simulink model "faultSimulation"  (R2024a)
settings: Solver=VariableStepAuto  StartTime=0.0  StopTime=0.5  RelTol=1e-3
libraries: spsThreePhaseVIMeasurementLib x2, spsRMSLib x2, spsDistributedParametersLineLib x2, spsSequenceAnalyzerLib x2, spsThreePhaseSeriesRLCLoadLib x1, spsThreePhaseSourceLib x1, spsThreePhaseTransformerTwoWindingsLib x1, spsThreePhaseFaultLib x1, spspowerguiLib x1
settings Model: Creator=Subash  LastModifiedBy=subed
settings DataIOCC: SaveFormat=StructureWithTime  SaveState=on  ReturnWorkspaceOutputs=off
settings OptimizationCC: ReuseModelBlockBuffer=off
settings RTWCC: GPUComputeCapability=3.5

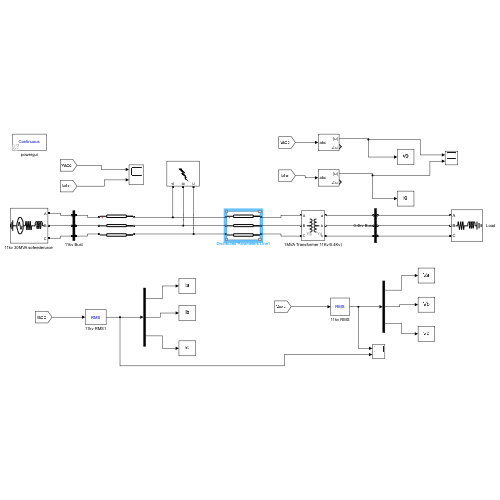
[thumbnail: Simulink's stored preview of the top-level diagram]
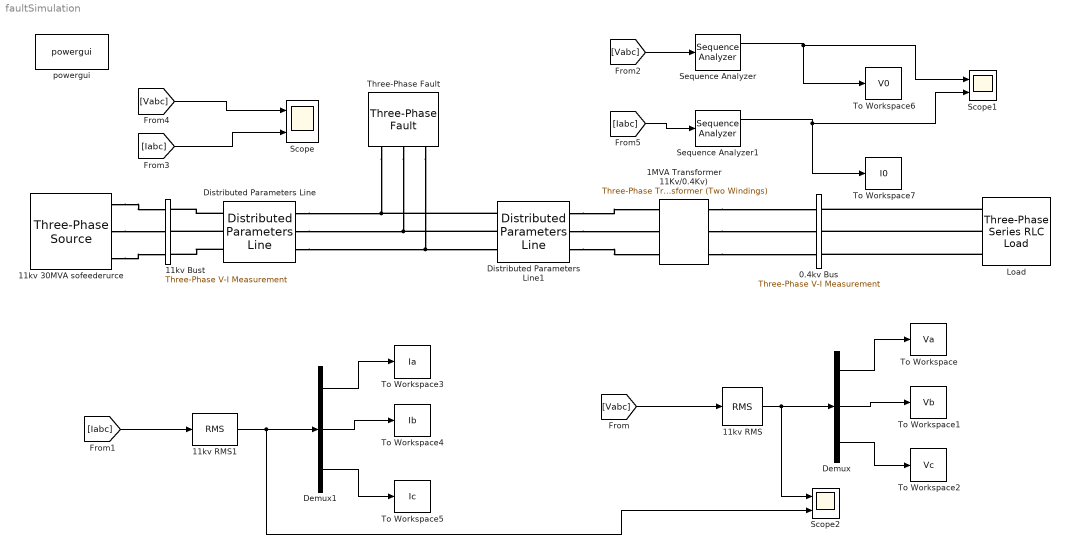
== system faultSimulation ==
  " Load" : spsThreePhaseSeriesRLCLoadLib/Three-Phase Series RLC Load  LConnTagsString=A|B|C  Configuration=Y (grounded)  NominalVoltage=11000  Vabc=[1e3 1e3 1e3]  Vabcp=[1e3 1e3 1e3]  NominalFrequency=50  UnbalancedPower=off  ActivePower=11e3  InductivePower=1  CapacitivePower=0  Pabc=[10e3 9e3 11e3]  QLabc=[100 90 110]  QCabc=0  Pabcp=[10e3 9e3 11e3]  QLabcp=[100 90 110]  QCabcp=[100 90 110]  Measurements=None  LoadType=constant Z
  0.4kv Bus : spsThreePhaseVIMeasurementLib/Three-Phase V-I Measurement  VoltageMeasurement=no  SetLabelV=off  LabelV=Vabc  Vpu=off  VpuLL=off  CurrentMeasurement=no  SetLabelI=off  LabelI=Iabc  Ipu=off  Pbase=100e6  Vbase=500e3  OutputType=Complex  PhasorSimulation=off  PSBequivalent=0
  "11kv 30MVA sofeederurce " : spsThreePhaseSourceLib/Three-Phase Source  InternalConnection=Yg  VoltagePhases=off  Voltage=11e3  PhaseAngle=0  Voltage_phases=[25e3 25e3 25e3]/sqrt(3)  PhaseAngles_phases=[0 -120 +120]  Frequency=50  NonIdealSource=on  SpecifyImpedance=off  Resistance=0.8929  Inductance=16.58e-3  ShortCircuitLevel=100e6  BaseVoltage=25e3  XRratio=7  BusType=PV  Pref=30e6  Qref=0  Prefabc=[10e3, 10e3, 10e3]  Qrefabc=[0, 0, 0]  Qmin=-inf  Qmax=inf
  11kv Bust : spsThreePhaseVIMeasurementLib/Three-Phase V-I Measurement  VoltageMeasurement=phase-to-ground  SetLabelV=on  LabelV=Vabc  Vpu=off  VpuLL=off  CurrentMeasurement=yes  SetLabelI=on  LabelI=Iabc  Ipu=off  Pbase=100e6  Vbase=500e3  OutputType=Complex  PhasorSimulation=off  PSBequivalent=0
  11kv RMS : spsRMSLib/RMS  TrueRMS=on  Freq=50  RMSInit=11e3  Ts=0
  11kv RMS1 : spsRMSLib/RMS  TrueRMS=on  Freq=50  RMSInit=11e3  Ts=0
  1MVA Transformer 11Kv/0.4Kv) : spsThreePhaseTransformerTwoWindingsLib/Three-Phase Transformer (Two Windings)  Winding1Connection=Yg  Winding2Connection=Yg  CoreType=Three single-phase transformers  SetSaturation=off  Hysteresis=off  DataFile='hysteresis'  SetInitialFlux=off  Measurements=None  UNITS=pu  NominalPower=[ 250e6 , 50 ]  Winding1=[ 11e3 , 0.002 , 0.08 ]  Winding2=[ 0.4e3 , 0.002 , 0.08 ]  Rm=500  Lm=500  L0=0.5  Saturation=[ 0,0 ; 0.0024,1.2 ; 1.0,1.52 ]  InitialFluxes=[0.8 -0.8 0.69999]  BreakLoop=off  DiscreteSolver=Trapezoidal iterative  DataType=off  TransfoNumber=1
  Demux : Demux  Outputs=3
  Demux1 : Demux  Outputs=3
  Distributed Parameters Line : spsDistributedParametersLineLib/Distributed Parameters Line  Phases=3  Length=10  Frequency=50  Resistance=[0.01273 0.3864]  Inductance="[0.9337e-3  4.1264e-3]"  Capacitance=[12.74e-9 7.751e-9]  x1=[4.29007792811563e-12 11003.1893836905 11003.1893836905;314.159265358979 314.159265358979 314.159265358979;2.11162862981672 0.512613974625824 -1.05818235216907]  x2=[2.73605273041382e-11 11004.416576192 11004.416576192;314.159265358979 314.159265358979 314.159265358979;2.85465814848236 0.512554423166818 -1.05824190362808]  x3=[2.29013626664532e-12 40.4303240016951 40.430324001691;314.159265358979 314.159265358979 314.159265358979;1.52130621419638 0.496602964655876 -1.07419336213898]  x4=[1.63728049127687e-12 40.8398210682543 40.8398210682578;314.159265358979 314.159265358979 314.159265358979;-1.19077244951278 0.517623004877797 -1.05317332191716]  x5=5.65541566995743e-05  V1=[4.29e-12 1.1e+04 1.1e+04;314.2 314.2 314.2;2.112 0.5126 -1.058]  V2=[2.736e-11 1.1e+04 1.1e+04;314.2 314.2 314.2;2.855 0.5126 -1.058]  I1=[2.29e-12 40.43 40.43;314.2 314.2 314.2;1.521 0.4966 -1.074]  I2=[1.637e-12 40.84 40.84;314.2 314.2 314.2;-1.191 0.5176 -1.053]  nHarmo=1  Measurements=None  Decoupling=off  VsMag0=0  VrMag0=0  VsAngle0=0  VrAngle0=0  IsMag0=0  IrMag0=0  IsAngle0=0  IrAngle0=0
      settings: LibrarySourceBlock=sps_lib/Power Grid Elements/Distributed Parameters Line
  Distributed Parameters Line1 : spsDistributedParametersLineLib/Distributed Parameters Line  Phases=3  Length=15  Frequency=50  Resistance=[0.01273 0.3864]  Inductance="[0.9337e-3  4.1264e-3]"  Capacitance=[12.74e-9 7.751e-9]  x1=[2.73605273041382e-11 11004.416576192 11004.416576192;314.159265358979 314.159265358979 314.159265358979;2.86354165464323 0.517972039807862 -1.05282428698704]  x2=[2.80656861363413e-11 11004.5464151717 11004.5464151717;314.159265358979 314.159265358979 314.159265358979;2.66181528844822 0.51794564452879 -1.05285068226611]  x3=[1.0173475413593e-12 40.4483736960803 40.4483736960805;314.159265358979 314.159265358979 314.159265358979;-2.35891284635151 0.512853803783494 -1.05794252301145]  x4=[1.45823347498536e-12 40.8359622190735 40.8359622190726;314.159265358979 314.159265358979 314.159265358979;3.13298239483697 0.517623203319764 -1.05317312347505]  x5=2.82770783497871e-05  V1=[2.736e-11 1.1e+04 1.1e+04;314.2 314.2 314.2;2.864 0.518 -1.053]  V2=[2.807e-11 1.1e+04 1.1e+04;314.2 314.2 314.2;2.662 0.5179 -1.053]  I1=[1.017e-12 40.45 40.45;314.2 314.2 314.2;-2.359 0.5129 -1.058]  I2=[1.458e-12 40.84 40.84;314.2 314.2 314.2;3.133 0.5176 -1.053]  nHarmo=1  Measurements=None  Decoupling=off  VsMag0=0  VrMag0=0  VsAngle0=0  VrAngle0=0  IsMag0=0  IrMag0=0  IsAngle0=0  IrAngle0=0
      settings: LibrarySourceBlock=sps_lib/Power Grid Elements/Distributed Parameters Line
  Scope : Scope  NumInputPorts=2
  Scope1 : Scope  NumInputPorts=2
  Scope2 : Scope  NumInputPorts=2
  Sequence Analyzer : spsSequenceAnalyzerLib/Sequence Analyzer  Freq=50  n=1  seq=Zero  InInit=[1, 0]  Ts=0
      settings: LibrarySourceBlock=sps_lib/Sensors and Measurements/Sequence Analyzer
  Sequence Analyzer1 : spsSequenceAnalyzerLib/Sequence Analyzer  Freq=50  n=1  seq=Zero  InInit=[1, 0]  Ts=0
      settings: LibrarySourceBlock=sps_lib/Sensors and Measurements/Sequence Analyzer
  Three-Phase Fault : spsThreePhaseFaultLib/Three-Phase Fault  InitialStates=0  FaultA=on  FaultB=off  FaultC=off  GroundFault=on  SwitchTimes=[0.2 0.3]  External=off  SwitchStatus=NaN  FaultResistance=0.001  GroundResistance=0.01  SnubberResistance=1e6  SnubberCapacitance=inf  Measurements=Fault voltages and currents
  To Workspace : ToWorkspace  VariableName=Va  SampleTime=-1
      settings: MaxDataPoints=15
  To Workspace1 : ToWorkspace  VariableName=Vb  SampleTime=-1
      settings: MaxDataPoints=15
  To Workspace2 : ToWorkspace  VariableName=Vc  SampleTime=-1
      settings: MaxDataPoints=15
  To Workspace3 : ToWorkspace  VariableName=Ia  SampleTime=-1
      settings: MaxDataPoints=15
  To Workspace4 : ToWorkspace  VariableName=Ib  SampleTime=-1
      settings: MaxDataPoints=15
  To Workspace5 : ToWorkspace  VariableName=Ic  SampleTime=-1
      settings: MaxDataPoints=15
  To Workspace6 : ToWorkspace  VariableName=V0  SampleTime=-1
      settings: MaxDataPoints=15
  To Workspace7 : ToWorkspace  VariableName=I0  SampleTime=-1
      settings: MaxDataPoints=15
  powergui : spspowerguiLib/powergui  Priority=1  SimulationMode=Continuous  SampleTime=50e-6  frequency=60  Iterations=50  frequencyindice=50  Pbase=100e6  ErrMax=1e-4  UnitsV=kV  UnitsW=MW  buscounter=0  FunctionMessages=off  echomessages=off  EnableUseOfTLC=off  CurrentSourceSwitches=off  DisableSnubberDevices=off  DisableRonSwitches=off  DisableVfSwitches=off  DisplayEquations=off  AutomaticDiscreteSolvers=off  SolverType=Tustin/Backward Euler (TBE)  Interpol=off  ExternalGateDelay=off  methode=off  Ts=100  x0status=blocks  SPID=on  SwTol=0  HookPort=off  NonlinearTolerance=1e-4  nMaxIteration=100  ContinueOnMaxIteration=off  RestoreLinks=warning  ResistiveCurrentMeasurement=off  Frange=[0:2:500]  Ylog=off  Xlog=on  ShowGrid=off  save=off  variable=ZData  structure=0  ZoomFFT=off  StartTime=0.0  cycles=1  DisplayStyle=1  fundamental=60  FreqAxis=off  MaxFrequency=1000  frequencyindicesteady=1  RmsSteady=1  display=off
  wires:
  Sequence Analyzer1/1 -> Scope1/2, To Workspace7/1
  [Iabc] -> Scope/2
  [Vabc] -> Scope/1
  Demux/2 -> To Workspace1/1
  Demux1/3 -> To Workspace5/1
  Demux/3 -> To Workspace2/1
  11kv RMS1/1 -> Scope2/2, Demux1/1
  11kv RMS/1 -> Scope2/1, Demux/1
  Demux/1 -> To Workspace/1
  Demux1/1 -> To Workspace3/1
  Demux1/2 -> To Workspace4/1
  Sequence Analyzer/1 -> Scope1/1, To Workspace6/1
  [Vabc] -> Sequence Analyzer/1
  [Iabc] -> 11kv RMS1/1
  [Vabc] -> 11kv RMS/1
  [Iabc] -> Sequence Analyzer1/1
  connections:
  Three-Phase Fault/LConn3 -- Distributed Parameters Line1/LConn3 -- Distributed Parameters Line/RConn3
  Distributed Parameters Line/RConn1 -- Distributed Parameters Line1/LConn1 -- Three-Phase Fault/LConn1
  Three-Phase Fault/LConn2 -- Distributed Parameters Line1/LConn2 -- Distributed Parameters Line/RConn2
  " Load"/LConn2 -- 0.4kv Bus/RConn2
  Distributed Parameters Line/LConn3 -- 11kv Bust/RConn3
  " Load"/LConn1 -- 0.4kv Bus/RConn1
  "11kv 30MVA sofeederurce "/RConn1 -- 11kv Bust/LConn1
  Distributed Parameters Line1/RConn1 -- 1MVA Transformer 11Kv/0.4Kv)/LConn1
  Distributed Parameters Line/LConn1 -- 11kv Bust/RConn1
  Distributed Parameters Line/LConn2 -- 11kv Bust/RConn2
  "11kv 30MVA sofeederurce "/RConn2 -- 11kv Bust/LConn2
  Distributed Parameters Line1/RConn2 -- 1MVA Transformer 11Kv/0.4Kv)/LConn2
  1MVA Transformer 11Kv/0.4Kv)/RConn3 -- 0.4kv Bus/LConn3
  " Load"/LConn3 -- 0.4kv Bus/RConn3
  1MVA Transformer 11Kv/0.4Kv)/RConn2 -- 0.4kv Bus/LConn2
  Distributed Parameters Line1/RConn3 -- 1MVA Transformer 11Kv/0.4Kv)/LConn3
  "11kv 30MVA sofeederurce "/RConn3 -- 11kv Bust/LConn3
  1MVA Transformer 11Kv/0.4Kv)/RConn1 -- 0.4kv Bus/LConn1
